simulink model "real_hengce_onlyname"  (R2012b)
settings: Solver=ode1  SolverMode=SingleTasking  StartTime=0.0  StopTime=inf  FixedStep=0.005  RelTol=1e-3
settings Model: SimulationMode=external  ExtModeTrigDuration=200000  Creator=5420  LastModifiedBy=Administrator
settings DataIOCC: SignalLoggingSaveFormat=ModelDataLogs  SignalLoggingName=sigsOut
settings OptimizationCC: InitFltsAndDblsToZero=on
settings DebuggingCC: SaveWithParameterizedLinksMsg=none  SignalResolutionControl=TryResolveAllWithWarning  SolverPrmCheckMsg=none  MultiTaskDSMMsg=warning  MultiTaskCondExecSysMsg=none  StrictBusMsg=None
settings RTWCC: SystemTargetFile=rtwin.tlc  TemplateMakefile=rtwin.tmf  Description=Real-Time Windows Target  ProcessScript=rtwin_make_rtw_hook  IncludeERTFirstTime=on
settings RTWinTargetCC: TargetFcnLib=ansi_tfl_tmw.mat  TargetLibSuffix=_rtwin.lib  TargetPreCompLibLocation=C:\Program Files\MATLAB\R2012b\toolbox\rtw\targets\rtwin\lib\win32  CodeReplacementLibrary=ANSI_C  ModelReferenceCompliant=off  CompOptLevelCompliant=off  RTWinDir=C:/PROGRA~1/MATLAB/R2012b/toolbox/rtw/targets/rtwin  TargetArch=win32

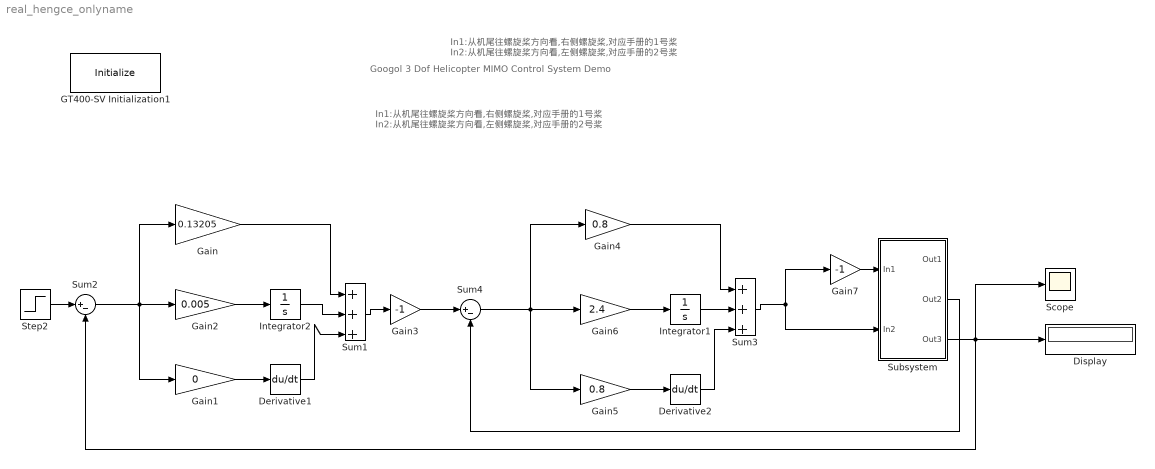
== system real_hengce_onlyname ==
  note: Googol 3 Dof Helicopter MIMO Control System Demo
  note: In1:从机尾往螺旋桨方向看,右侧螺旋桨,对应手册的1号桨
      | In2:从机尾往螺旋桨方向看,左侧螺旋桨,对应手册的2号桨
  note: In1:从机尾往螺旋桨方向看,右侧螺旋桨,对应手册的1号桨
      | In2:从机尾往螺旋桨方向看,左侧螺旋桨,对应手册的2号桨
  Derivative1 : Derivative
  Derivative2 : Derivative
  Display : Display
  GT400-SV Initialization1 : S-Function  Priority=0  FunctionName=Initialize  Parameters=openloop  EnableBusSupport=off  mask(Initialize){openloop=1}
      mask prompts: openloop "Control loop:"
      mask help:
      | Initializing the googol GT400-SV motion control board.
      | Block parameter:
      |     Control loop:
      |          0: closed-loop control.
      |          1: opened-loop control.
      mask Help: This initialize block initializes the googol GT400-SV motion control board.
      mask Display: disp('Initialize \nGT400-SV');
  Gain : Gain  Gain=0.13205
  Gain1 : Gain  Gain=0
  Gain2 : Gain  Gain=0.005
  Gain3 : Gain  Gain=-1
  Gain4 : Gain  Gain=0.8
  Gain5 : Gain  Gain=0.8
  Gain6 : Gain  Gain=2.4
  Gain7 : Gain  Gain=-1
  Integrator1 : Integrator
  Integrator2 : Integrator
  Scope : Scope
      settings: MaxDataPoints=500000
  Step2 : Step  After=3.14  SampleTime=0
  Subsystem : Subsystem
  Sum1 : Sum  Inputs=|+++
  Sum2 : Sum  Inputs=|+-
  Sum3 : Sum  Inputs=|+++
  Sum4 : Sum  Inputs=|+-
  wires:
  Integrator2/1 -> Sum1/2
  Derivative1/1 -> Sum1/3
  Gain1/1 -> Derivative1/1
  Gain2/1 -> Integrator2/1
  Step2/1 -> Sum2/1
  Sum2/1 -> Gain1/1, Gain/1, Gain2/1
  Sum1/1 -> Gain3/1
  Gain/1 -> Sum1/1
  Integrator1/1 -> Sum3/2
  Derivative2/1 -> Sum3/3
  Gain5/1 -> Derivative2/1
  Gain6/1 -> Integrator1/1
  Gain4/1 -> Sum3/1
  Gain3/1 -> Sum4/1
  Sum4/1 -> Gain5/1, Gain6/1, Gain4/1
  Sum3/1 -> Subsystem/2(In2), Gain7/1
  Gain7/1 -> Subsystem/1(In1)
  Subsystem/3(Out3) -> Sum2/2, Display/1, Scope/1
  Subsystem/2(Out2) -> Sum4/2

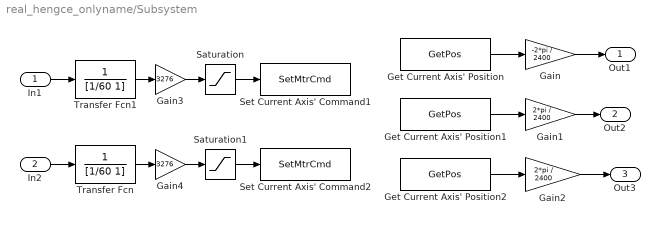
== system real_hengce_onlyname/Subsystem ==
  In1 : Inport
  In2 : Inport  Port=2
  Gain : Gain  Gain=-2*pi / 2400  SaturateOnIntegerOverflow=on  OutDataTypeStr=Inherit: Same as input  ParamDataTypeStr=Inherit: Same as input
  Gain1 : Gain  Gain=2*pi / 2400  SaturateOnIntegerOverflow=on  OutDataTypeStr=Inherit: Same as input  ParamDataTypeStr=Inherit: Same as input
  Gain2 : Gain  Gain=2*pi / 2400  SaturateOnIntegerOverflow=on  OutDataTypeStr=Inherit: Same as input  ParamDataTypeStr=Inherit: Same as input
  Gain3 : Gain  Gain=3276
  Gain4 : Gain  Gain=3276
  Get Current Axis' Position : S-Function  Priority=1  FunctionName=GetPos  Parameters=axis  EnableBusSupport=off  mask(GetPos){axis=2}
      mask prompts: axis "Axis number:"
      mask help:
      | Getting the current axis position value in encoder' counts.
      | Block parameter:
      |     Axis number:  must be between 1 and 6, default is 1.
      | Block output:
      |     1~4: current axis' encoder reading counts.
      |     5/6: assistant encoder 1/2 reading counts.
      mask Help:
      | This block, GetPos, is intended for getting the current axis position value in encoder' counts. This value represents the actual position for the axis
      | at the current sample time. This command operates for all profile modes.
      | The value returned is a 32-bit signed number with units of counts.
      | The range is -1,073,741,824 to 1,073,741,823.
      | 
      | You can recalculate obtained value into meter units via multiplication by the scaler coefficient .
      | 
      | Block parameter:
      |     Axis number:  must be between 1 and 4, default is 1.
      | Block input: none.
      | Block output:
      |         1~4: current axis' encoder reading counts.
      |         5/6: assistant encoder 1/2 reading counts.
      mask Display:
      | disp('GetPos');
      | port_label('output', 1, 'Pos');
  Get Current Axis' Position1 : S-Function  Priority=1  FunctionName=GetPos  Parameters=axis  EnableBusSupport=off  mask(GetPos){axis=1}
      mask prompts: axis "Axis number:"
      mask help:
      | Getting the current axis position value in encoder' counts.
      | Block parameter:
      |     Axis number:  must be between 1 and 6, default is 1.
      | Block output:
      |     1~4: current axis' encoder reading counts.
      |     5/6: assistant encoder 1/2 reading counts.
      mask Help:
      | This block, GetPos, is intended for getting the current axis position value in encoder' counts. This value represents the actual position for the axis
      | at the current sample time. This command operates for all profile modes.
      | The value returned is a 32-bit signed number with units of counts.
      | The range is -1,073,741,824 to 1,073,741,823.
      | 
      | You can recalculate obtained value into meter units via multiplication by the scaler coefficient .
      | 
      | Block parameter:
      |     Axis number:  must be between 1 and 4, default is 1.
      | Block input: none.
      | Block output:
      |         1~4: current axis' encoder reading counts.
      |         5/6: assistant encoder 1/2 reading counts.
      mask Display:
      | disp('GetPos');
      | port_label('output', 1, 'Pos');
  Get Current Axis' Position2 : S-Function  Priority=1  FunctionName=GetPos  Parameters=axis  EnableBusSupport=off  mask(GetPos){axis=3}
      mask prompts: axis "Axis number:"
      mask help:
      | Getting the current axis position value in encoder' counts.
      | Block parameter:
      |     Axis number:  must be between 1 and 6, default is 1.
      | Block output:
      |     1~4: current axis' encoder reading counts.
      |     5/6: assistant encoder 1/2 reading counts.
      mask Help:
      | This block, GetPos, is intended for getting the current axis position value in encoder' counts. This value represents the actual position for the axis
      | at the current sample time. This command operates for all profile modes.
      | The value returned is a 32-bit signed number with units of counts.
      | The range is -1,073,741,824 to 1,073,741,823.
      | 
      | You can recalculate obtained value into meter units via multiplication by the scaler coefficient .
      | 
      | Block parameter:
      |     Axis number:  must be between 1 and 4, default is 1.
      | Block input: none.
      | Block output:
      |         1~4: current axis' encoder reading counts.
      |         5/6: assistant encoder 1/2 reading counts.
      mask Display:
      | disp('GetPos');
      | port_label('output', 1, 'Pos');
  Saturation : Saturate  UpperLimit=9000  LowerLimit=0
  Saturation1 : Saturate  UpperLimit=9000  LowerLimit=0
  Set Current Axis' Command1 : S-Function  Priority=1  FunctionName=SetMtrCmd  Parameters=axis  EnableBusSupport=off  mask(SetMtrCmd){axis=1}
      mask prompts: axis "Axis number:"
      mask help:
      | Settting the current axis' voltage.
      | Block parameter:
      |     Axis number:  must be between 1 and 4, default is 1.
      | Block input:
      |     the current axis' voltage.
      mask Help:
      | This SetMtrCmd settting the current axis' voltage.
      | Block parameter:
      |     Axis number:  must be between 1 and 4, default is 1.
      mask Display:
      | disp('          SetMtrCmd');
      | port_label('input', 1, 'Vol');
  Set Current Axis' Command2 : S-Function  Priority=1  FunctionName=SetMtrCmd  Parameters=axis  EnableBusSupport=off  mask(SetMtrCmd){axis=2}
      mask prompts: axis "Axis number:"
      mask help:
      | Settting the current axis' voltage.
      | Block parameter:
      |     Axis number:  must be between 1 and 4, default is 1.
      | Block input:
      |     the current axis' voltage.
      mask Help:
      | This SetMtrCmd settting the current axis' voltage.
      | Block parameter:
      |     Axis number:  must be between 1 and 4, default is 1.
      mask Display:
      | disp('          SetMtrCmd');
      | port_label('input', 1, 'Vol');
  Transfer Fcn : TransferFcn  Denominator=[1/60 1]
  Transfer Fcn1 : TransferFcn  Denominator=[1/60 1]
  Out1 : Outport
  Out2 : Outport  Port=2
  Out3 : Outport  Port=3
  wires:
  Get Current Axis' Position/1 -> Gain/1
  Get Current Axis' Position1/1 -> Gain1/1
  Get Current Axis' Position2/1 -> Gain2/1
  Gain/1 -> Out1/1
  Gain1/1 -> Out2/1
  Gain2/1 -> Out3/1
  In2/1 -> Transfer Fcn/1
  In1/1 -> Transfer Fcn1/1
  Gain3/1 -> Saturation/1
  Saturation/1 -> Set Current Axis' Command1/1
  Gain4/1 -> Saturation1/1
  Saturation1/1 -> Set Current Axis' Command2/1
  Transfer Fcn/1 -> Gain4/1
  Transfer Fcn1/1 -> Gain3/1
